simulink model "Test_N5"  (R2022a)
settings: Solver=ode3  StartTime=0.0  StopTime=inf  FixedStep=0.05  RelTol=1e-3
libraries: EcBlockToolbox x1

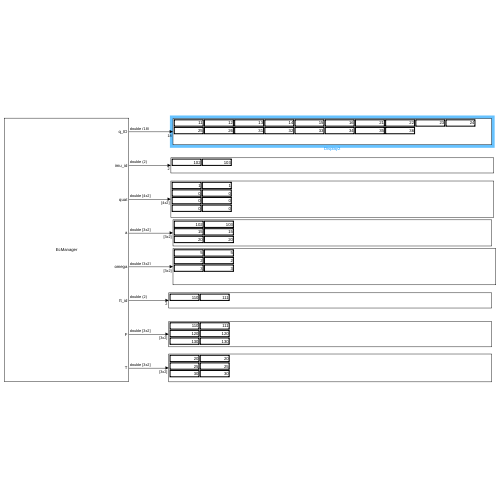
[thumbnail: Simulink's stored preview of the top-level diagram]
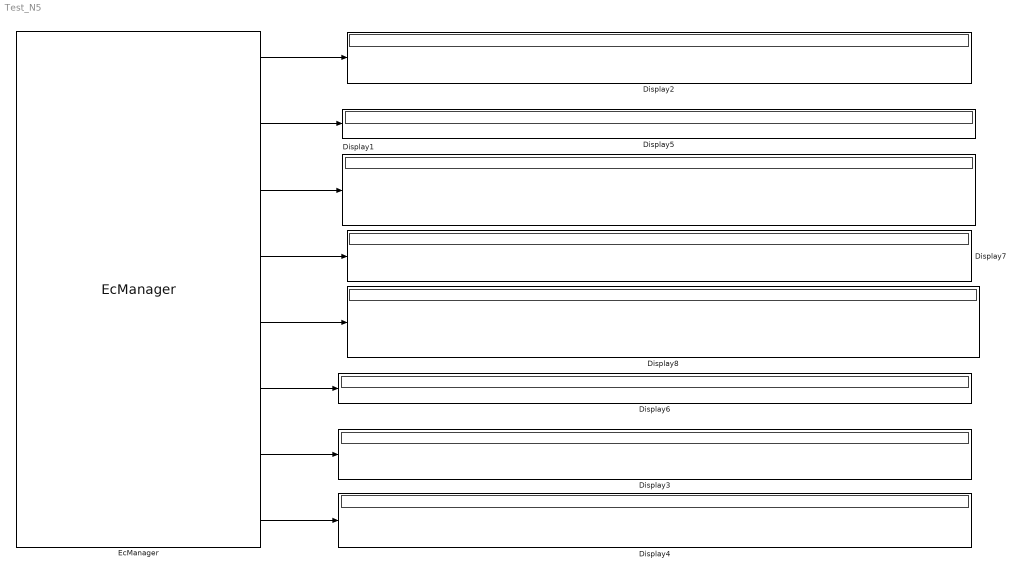
== system Test_N5 ==
  Display{1..8} (8 alike) : Display
  EcManager : EcBlockToolbox/EcManager  ReadingsList={'q_ID'}  ReferencesList={}  ImuList={'imu_id', 'quat', 'a', 'omega'}  FtList={'ft_id', 'F', 'T'}
  wires:
  EcManager/8 -> Display4/1
  EcManager/1 -> Display2/1
  EcManager/3 -> Display1/1
  EcManager/7 -> Display3/1
  EcManager/2 -> Display5/1
  EcManager/6 -> Display6/1
  EcManager/4 -> Display7/1
  EcManager/5 -> Display8/1
